simulink model "mrefrobotarm_modified_previous_y_previous_u_previous_ref"  (R2018b)
settings: Solver=FixedStepAuto  StartTime=0.0  StopTime=10  RelTol=1e-3  AbsTol=1e-6
undefined symbols (not defined in the file or in its folder): options, sfunxy2
libraries: neural x949, simulink x1
(part 22 of 31)

== system mrefrobotarm_modified_previous_y_previous_u_previous_ref/const_51traces_30x30_σ_0.0001/Layer 3/Delays 1 ==
  "p{3}" : Inport  PortDimensions=30
      mask Display: e = 0.06;c1 = [120 230 180]/255;c2 = ([120 230 180]+0)/(256+128);c3 = ([120 230 180]+128)/(256+128);patch([0 1 1 0],[0 0 1 1],c1);patch([0 1 1 1-e 1-e 0+e],[0 0 1 1-e 0+e 0+e],c2);patch([0 0 1 1-e 0+e 0+e],[0 1 1 1-e 1-e 0+e],c3);plot([0 1 1 0 0],[0 0 1 1 0]);
  mux : Mux  Inputs=1
      mask Display: e = 0.06;c1 = [120 150 230]/255;c2 = ([120 150 230]+0)/383;c3 = ([120 150 230]+128)/383;patch([0 1 1 0],[0 0 1 1],c1);patch([0 1 1 1-e 1-e 0+e],[0 0 1 1-e 0+e 0+e],c2);patch([0 0 1 1-e 0+e 0+e],[0 1 1 1-e 1-e 0+e],c3);plot([0 1 1 0 0],[0 0 1 1 0]);disp('Mux')
  "pd{3,2}" : Outport
      mask Display: e = 0.06;c1 = [120 230 180]/255;c2 = ([120 230 180]+0)/(256+128);c3 = ([120 230 180]+128)/(256+128);patch([0 1 1 0],[0 0 1 1],c1);patch([0 1 1 1-e 1-e 0+e],[0 0 1 1-e 0+e 0+e],c2);patch([0 0 1 1-e 0+e 0+e],[0 1 1 1-e 1-e 0+e],c3);plot([0 1 1 0 0],[0 0 1 1 0]);
  wires:
  "p{3}"/1 -> mux/1
  mux/1 -> "pd{3,2}"/1

== system mrefrobotarm_modified_previous_y_previous_u_previous_ref/const_51traces_30x30_σ_0.0001/Layer 3/LW{3,2} ==
  "ad{3,2}" : Inport  PortDimensions=30
      mask Display: e = 0.06;c1 = [120 230 180]/255;c2 = ([120 230 180]+0)/(256+128);c3 = ([120 230 180]+128)/(256+128);patch([0 1 1 0],[0 0 1 1],c1);patch([0 1 1 1-e 1-e 0+e],[0 0 1 1-e 0+e 0+e],c2);patch([0 0 1 1-e 0+e 0+e],[0 1 1 1-e 1-e 0+e],c3);plot([0 1 1 0 0],[0 0 1 1 0]);
  "IW{3,2}(1,:)'" : Constant  Value=[0.240977023629920295011430653175921179354190826416015625;-0.72988152363239200415279128719703294336795806884765625;-0.0304462107496987245680575284723090589977800846099853515625;-0.635040700178726158497966025606729090213775634765625;-0.612453231448408796921967223170213401317596435546875;-0.1344363308878322171846519950122456066310405731201171875;0.432506655045428123340656156869954429566860198974609375;-0.176669851226666951848898179378011263906955718994140625;-0.07557040530097362818207074042220483534038066864013671875;-0.41772110776708348822694460977800190448760986328125;0.93149781158754973997560000498197041451930999755859375;-0.31563700822511797650093967604334466159343719482421875;0.179588162001579565441033992101438343524932861328125;0.367943037247817239521197052454226650297641754150390625;0.41883849740428102936817822410375811159610748291015625;-0.50851554248389507772998285872745327651500701904296875;0.230395821119363464202223212851095013320446014404296875;-0.57517747958286757903323405116680078208446502685546875;0.71954478083832607016034899061196483671665191650390625;0.42048070720552555012972106851520948112010955810546875;-0.6720740263233346833970927036716602742671966552734375;0.183028758641015365515869461887632496654987335205078125;-0.25324226100094671121354394927038811147212982177734375;-0.0872596554170980975850824279405060224235057830810546875;-0.2750454559251604980119054744136519730091094970703125;-0.576829150618785480020278555457480251789093017578125;0.86151412289092366147968959921854548156261444091796875;-0.6458765000689965507518763843108899891376495361328125;1.0786071922365649822239674904267303645610809326171875;0.399731589161183453740022741840220987796783447265625]
      mask Display: e = 0.06;c1 = [120 150 230]/255;c2 = ([120 150 230]+0)/383;c3 = ([120 150 230]+128)/383;patch([0 1 1 0],[0 0 1 1],c1);patch([0 1 1 1-e 1-e 0+e],[0 0 1 1-e 0+e 0+e],c2);patch([0 0 1 1-e 0+e 0+e],[0 1 1 1-e 1-e 0+e],c3);plot([0 1 1 0 0],[0 0 1 1 0]);disp('weights');
  Mux : Mux  Inputs=1
      mask Display: e = 0.06;c1 = [120 150 230]/255;c2 = ([120 150 230]+0)/383;c3 = ([120 150 230]+128)/383;patch([0 1 1 0],[0 0 1 1],c1);patch([0 1 1 1-e 1-e 0+e],[0 0 1 1-e 0+e 0+e],c2);patch([0 0 1 1-e 0+e 0+e],[0 1 1 1-e 1-e 0+e],c3);plot([0 1 1 0 0],[0 0 1 1 0]);disp('Mux');
  dotprod1 : neural/Weight Functions/dotprod
  "lz{3,2}" : Outport
      mask Display: e = 0.06;c1 = [120 230 180]/255;c2 = ([120 230 180]+0)/(256+128);c3 = ([120 230 180]+128)/(256+128);patch([0 1 1 0],[0 0 1 1],c1);patch([0 1 1 1-e 1-e 0+e],[0 0 1 1-e 0+e 0+e],c2);patch([0 0 1 1-e 0+e 0+e],[0 1 1 1-e 1-e 0+e],c3);plot([0 1 1 0 0],[0 0 1 1 0]);
  wires:
  "IW{3,2}(1,:)'"/1 -> dotprod1/1
  "ad{3,2}"/1 -> dotprod1/2
  dotprod1/1 -> Mux/1
  Mux/1 -> "lz{3,2}"/1

== system mrefrobotarm_modified_previous_y_previous_u_previous_ref/const_51traces_30x30_σ_0.001/Layer 1/Delays 1 ==
  "p{1}" : Inport  PortDimensions=10
      mask Display: e = 0.06;c1 = [120 230 180]/255;c2 = ([120 230 180]+0)/(256+128);c3 = ([120 230 180]+128)/(256+128);patch([0 1 1 0],[0 0 1 1],c1);patch([0 1 1 1-e 1-e 0+e],[0 0 1 1-e 0+e 0+e],c2);patch([0 0 1 1-e 0+e 0+e],[0 1 1 1-e 1-e 0+e],c3);plot([0 1 1 0 0],[0 0 1 1 0]);
  mux : Mux  Inputs=1
      mask Display: e = 0.06;c1 = [120 150 230]/255;c2 = ([120 150 230]+0)/383;c3 = ([120 150 230]+128)/383;patch([0 1 1 0],[0 0 1 1],c1);patch([0 1 1 1-e 1-e 0+e],[0 0 1 1-e 0+e 0+e],c2);patch([0 0 1 1-e 0+e 0+e],[0 1 1 1-e 1-e 0+e],c3);plot([0 1 1 0 0],[0 0 1 1 0]);disp('Mux')
  "pd{1,1}" : Outport
      mask Display: e = 0.06;c1 = [120 230 180]/255;c2 = ([120 230 180]+0)/(256+128);c3 = ([120 230 180]+128)/(256+128);patch([0 1 1 0],[0 0 1 1],c1);patch([0 1 1 1-e 1-e 0+e],[0 0 1 1-e 0+e 0+e],c2);patch([0 0 1 1-e 0+e 0+e],[0 1 1 1-e 1-e 0+e],c3);plot([0 1 1 0 0],[0 0 1 1 0]);
  wires:
  "p{1}"/1 -> mux/1
  mux/1 -> "pd{1,1}"/1

== system mrefrobotarm_modified_previous_y_previous_u_previous_ref/const_51traces_30x30_σ_0.001/Layer 1/IW{1,1} ==
  "pd{1,1}" : Inport  PortDimensions=10
      mask Display: e = 0.06;c1 = [120 230 180]/255;c2 = ([120 230 180]+0)/(256+128);c3 = ([120 230 180]+128)/(256+128);patch([0 1 1 0],[0 0 1 1],c1);patch([0 1 1 1-e 1-e 0+e],[0 0 1 1-e 0+e 0+e],c2);patch([0 0 1 1-e 0+e 0+e],[0 1 1 1-e 1-e 0+e],c3);plot([0 1 1 0 0],[0 0 1 1 0]);
  "IW{1,1}(1,:)'" : Constant  Value=[0.88647590430992784238384274431155063211917877197265625;-1.14613055383974771217481247731484472751617431640625;0.43149650278918649792814221655135042965412139892578125;-0.3599801224142209488121579852304421365261077880859375;1.1960164258275838289335979425231926143169403076171875;-0.61109131411137285194712376323877833783626556396484375;-0.1400609285406480830626918532288982532918453216552734375;-0.5627127955935364855832858665962703526020050048828125;1.0868171814027147714654120136401616036891937255859375;0.590166554455455294458943171775899827480316162109375]
      mask Display: e = 0.06;c1 = [120 150 230]/255;c2 = ([120 150 230]+0)/383;c3 = ([120 150 230]+128)/383;patch([0 1 1 0],[0 0 1 1],c1);patch([0 1 1 1-e 1-e 0+e],[0 0 1 1-e 0+e 0+e],c2);patch([0 0 1 1-e 0+e 0+e],[0 1 1 1-e 1-e 0+e],c3);plot([0 1 1 0 0],[0 0 1 1 0]);disp('Weights');
  "IW{1,1}(10,:)'" : Constant  Value=[-1.2142966679649254135853198022232390940189361572265625;0.7923988402907820027820662289741449058055877685546875;-0.0939776780882374540571078114226111210882663726806640625;-0.43838558129977889255002310164854861795902252197265625;0.30510202260699303966617890182533301413059234619140625;0.0798827324582818409925977221064385958015918731689453125;-1.3502873847698875220402214836212806403636932373046875;-0.385994205104438770081998200112138874828815460205078125;-0.002611353880893824315478912723165194620378315448760986328125;0.5342263949565795311258398214704357087612152099609375]
      mask Display: e = 0.06;c1 = [120 150 230]/255;c2 = ([120 150 230]+0)/383;c3 = ([120 150 230]+128)/383;patch([0 1 1 0],[0 0 1 1],c1);patch([0 1 1 1-e 1-e 0+e],[0 0 1 1-e 0+e 0+e],c2);patch([0 0 1 1-e 0+e 0+e],[0 1 1 1-e 1-e 0+e],c3);plot([0 1 1 0 0],[0 0 1 1 0]);disp('Weights');
  "IW{1,1}(11,:)'" : Constant  Value=[0.52551988502623869781160692582488991320133209228515625;-1.3023156568469591576331367832608520984649658203125;-0.0716415511593599119155584276086301542818546295166015625;-0.55450379058502397011665152604109607636928558349609375;-0.230954917200865639248519300963380374014377593994140625;0.452249109231775470174596875949646346271038055419921875;-0.86426961935203916453929195995442569255828857421875;-0.9549970517556440885442725630127824842929840087890625;-0.1924050964451662071308390977719682268798351287841796875;0.10583122693447775952702016866169287823140621185302734375]
      mask Display: e = 0.06;c1 = [120 150 230]/255;c2 = ([120 150 230]+0)/383;c3 = ([120 150 230]+128)/383;patch([0 1 1 0],[0 0 1 1],c1);patch([0 1 1 1-e 1-e 0+e],[0 0 1 1-e 0+e 0+e],c2);patch([0 0 1 1-e 0+e 0+e],[0 1 1 1-e 1-e 0+e],c3);plot([0 1 1 0 0],[0 0 1 1 0]);disp('Weights');
  "IW{1,1}(12,:)'" : Constant  Value=[-0.387313692266497755500864741406985558569431304931640625;0.429686255286772678108064837942947633564472198486328125;-0.95932065522831300174999569208011962473392486572265625;-0.090550079651663784030546366921043954789638519287109375;0.5727868458286546893276636183145456016063690185546875;0.87868876198865553117656190806883387267589569091796875;-1.7317258283279617359085023053921759128570556640625;-0.8527971123216737669991971415583975613117218017578125;0.31308642872469338858110177170601673424243927001953125;0.372259712843441559204649138337117619812488555908203125]
      mask Display: e = 0.06;c1 = [120 150 230]/255;c2 = ([120 150 230]+0)/383;c3 = ([120 150 230]+128)/383;patch([0 1 1 0],[0 0 1 1],c1);patch([0 1 1 1-e 1-e 0+e],[0 0 1 1-e 0+e 0+e],c2);patch([0 0 1 1-e 0+e 0+e],[0 1 1 1-e 1-e 0+e],c3);plot([0 1 1 0 0],[0 0 1 1 0]);disp('Weights');
  "IW{1,1}(13,:)'" : Constant  Value=[-1.25614456387378492507878036121837794780731201171875;-0.5877910303392492874507979649933986365795135498046875;1.84758793112290931048846687190234661102294921875;-0.420507467934437217937926334343501366674900054931640625;-0.5430993843563971523735744995065033435821533203125;0.076738152362635203562746255556703545153141021728515625;-1.0783832881460242436588714554090984165668487548828125;0.0126228514731737927190291514989439747296273708343505859375;0.6739402421483422500614324235357344150543212890625;0.54534617577532717991317667838302440941333770751953125]
      mask Display: e = 0.06;c1 = [120 150 230]/255;c2 = ([120 150 230]+0)/383;c3 = ([120 150 230]+128)/383;patch([0 1 1 0],[0 0 1 1],c1);patch([0 1 1 1-e 1-e 0+e],[0 0 1 1-e 0+e 0+e],c2);patch([0 0 1 1-e 0+e 0+e],[0 1 1 1-e 1-e 0+e],c3);plot([0 1 1 0 0],[0 0 1 1 0]);disp('Weights');
  "IW{1,1}(14,:)'" : Constant  Value=[-0.5610919404950094335760013564140535891056060791015625;-0.054761539049275380353076769779363530687987804412841796875;1.42372282804068372996653124573640525341033935546875;-0.05361445587794340383869240440617431886494159698486328125;1.5687698740827966670252635594806633889675140380859375;-0.62361349109505581633783322104136459529399871826171875;0.281870101393739247441772022284567356109619140625;0.132740699085331648188201825178111903369426727294921875;-0.64733196498112566263927192267146892845630645751953125;-0.55118751847270852639582017218344844877719879150390625]
      mask Display: e = 0.06;c1 = [120 150 230]/255;c2 = ([120 150 230]+0)/383;c3 = ([120 150 230]+128)/383;patch([0 1 1 0],[0 0 1 1],c1);patch([0 1 1 1-e 1-e 0+e],[0 0 1 1-e 0+e 0+e],c2);patch([0 0 1 1-e 0+e 0+e],[0 1 1 1-e 1-e 0+e],c3);plot([0 1 1 0 0],[0 0 1 1 0]);disp('Weights');
  "IW{1,1}(15,:)'" : Constant  Value=[-1.9411344048006611284762357172439806163311004638671875;2.326146040891350796897540931240655481815338134765625;-0.230970377794815051597510091596632264554500579833984375;-0.0191512345205407281956144771584149566479027271270751953125;-0.05470523213543997120833495273473090492188930511474609375;-0.8832535760934174806635610366356559097766876220703125;1.1713944845459016708133503925637342035770416259765625;-0.405518430821696418409061379861668683588504791259765625;-0.1373891257194361503746193875485914759337902069091796875;-0.1887055562416380671830751225570566020905971527099609375]
      mask Display: e = 0.06;c1 = [120 150 230]/255;c2 = ([120 150 230]+0)/383;c3 = ([120 150 230]+128)/383;patch([0 1 1 0],[0 0 1 1],c1);patch([0 1 1 1-e 1-e 0+e],[0 0 1 1-e 0+e 0+e],c2);patch([0 0 1 1-e 0+e 0+e],[0 1 1 1-e 1-e 0+e],c3);plot([0 1 1 0 0],[0 0 1 1 0]);disp('Weights');
  "IW{1,1}(16,:)'" : Constant  Value=[-0.7164923870544532835680229254649020731449127197265625;-0.8690128499532681072281548040336929261684417724609375;0.331242213568548660163060048944316804409027099609375;0.476331520597255586579876762698404490947723388671875;-0.2392438611302276918468834310260717757046222686767578125;-1.648318417891640574879374980810098350048065185546875;0.6083784402561971393907924721133895218372344970703125;-0.479773713578626026521334324570489116013050079345703125;0.32137233228833517184597212690277956426143646240234375;-0.077657410543244598244427834288217127323150634765625]
      mask Display: e = 0.06;c1 = [120 150 230]/255;c2 = ([120 150 230]+0)/383;c3 = ([120 150 230]+128)/383;patch([0 1 1 0],[0 0 1 1],c1);patch([0 1 1 1-e 1-e 0+e],[0 0 1 1-e 0+e 0+e],c2);patch([0 0 1 1-e 0+e 0+e],[0 1 1 1-e 1-e 0+e],c3);plot([0 1 1 0 0],[0 0 1 1 0]);disp('Weights');
  "IW{1,1}(17,:)'" : Constant  Value=[-2.0928207094062347692897674278356134891510009765625;1.1333921124488590681522737213526852428913116455078125;0.2436558329696220936977368864972959272563457489013671875;0.57908718336795617087631171671091578900814056396484375;-0.053129695756825544294965624203541665337979793548583984375;0.82751060843652701759509682233328931033611297607421875;-0.7738951508536626722190021610003896057605743408203125;0.2119294387762725440094158102510846219956874847412109375;0.319819577337992988486092826860840432345867156982421875;0.251131352053680034774885143633582629263401031494140625]
      mask Display: e = 0.06;c1 = [120 150 230]/255;c2 = ([120 150 230]+0)/383;c3 = ([120 150 230]+128)/383;patch([0 1 1 0],[0 0 1 1],c1);patch([0 1 1 1-e 1-e 0+e],[0 0 1 1-e 0+e 0+e],c2);patch([0 0 1 1-e 0+e 0+e],[0 1 1 1-e 1-e 0+e],c3);plot([0 1 1 0 0],[0 0 1 1 0]);disp('Weights');
  "IW{1,1}(18,:)'" : Constant  Value=[-0.4122265323291178784614885444170795381069183349609375;0.73672628799896477946873574182973243296146392822265625;-0.239290661988695141371152885767514817416667938232421875;0.08962867920218543782429065913675003685057163238525390625;1.3130795126584458021312684650183655321598052978515625;0.8249569542701771229786800176952965557575225830078125;-0.5734716364476799554950048332102596759796142578125;0.32220931283260700883630534008261747658252716064453125;0.404090567428519176207402097134036011993885040283203125;0.402109996183113771461847818500245921313762664794921875]
      mask Display: e = 0.06;c1 = [120 150 230]/255;c2 = ([120 150 230]+0)/383;c3 = ([120 150 230]+128)/383;patch([0 1 1 0],[0 0 1 1],c1);patch([0 1 1 1-e 1-e 0+e],[0 0 1 1-e 0+e 0+e],c2);patch([0 0 1 1-e 0+e 0+e],[0 1 1 1-e 1-e 0+e],c3);plot([0 1 1 0 0],[0 0 1 1 0]);disp('Weights');
  "IW{1,1}(19,:)'" : Constant  Value=[-2.118850089708957273870737481047399342060089111328125;0.6347893845452656780281586179626174271106719970703125;0.97211407073288935709598490575444884598255157470703125;0.5121431870732011670810379655449651181697845458984375;-0.406246003226239216221671313178376294672489166259765625;0.94847719721738388276577325086691416800022125244140625;-0.7102564152048820300677789418841712176799774169921875;0.0811496480015026222520901910684187896549701690673828125;-0.077569687242050322506514703491120599210262298583984375;0.1878282976390456548987373253112309612333774566650390625]
      mask Display: e = 0.06;c1 = [120 150 230]/255;c2 = ([120 150 230]+0)/383;c3 = ([120 150 230]+128)/383;patch([0 1 1 0],[0 0 1 1],c1);patch([0 1 1 1-e 1-e 0+e],[0 0 1 1-e 0+e 0+e],c2);patch([0 0 1 1-e 0+e 0+e],[0 1 1 1-e 1-e 0+e],c3);plot([0 1 1 0 0],[0 0 1 1 0]);disp('Weights');
  "IW{1,1}(2,:)'" : Constant  Value=[-0.313257085634319254463520110220997594296932220458984375;0.7286897052037304423066643721540458500385284423828125;-0.5203645417886988422395688758115284144878387451171875;-0.51693659700237082343932115691131912171840667724609375;0.3651607836022439101952841156162321567535400390625;-0.64593850834349197942430009788949973881244659423828125;-0.336786483559425919853680397864081896841526031494140625;0.260117299543795976735083286257577128708362579345703125;-1.1992681308720600785733267912291921675205230712890625;-0.398556029791291288599808240178390406072139739990234375]
      mask Display: e = 0.06;c1 = [120 150 230]/255;c2 = ([120 150 230]+0)/383;c3 = ([120 150 230]+128)/383;patch([0 1 1 0],[0 0 1 1],c1);patch([0 1 1 1-e 1-e 0+e],[0 0 1 1-e 0+e 0+e],c2);patch([0 0 1 1-e 0+e 0+e],[0 1 1 1-e 1-e 0+e],c3);plot([0 1 1 0 0],[0 0 1 1 0]);disp('Weights');
  "IW{1,1}(20,:)'" : Constant  Value=[-2.325790065228988456880188095965422689914703369140625;-0.79385756422430109324750446830876171588897705078125;2.014777521227398171532740889233537018299102783203125;0.51980984727200529871282697058632038533687591552734375;-0.873647536591071638412131505901925265789031982421875;-0.297842745402778386054620796130620874464511871337890625;0.11769269572367714593585930060726241208612918853759765625;-0.009965195805270610218684623760054819285869598388671875;0.1877710921067496097069948746138834394514560699462890625;0.26877118123566756668907373750698752701282501220703125]
      mask Display: e = 0.06;c1 = [120 150 230]/255;c2 = ([120 150 230]+0)/383;c3 = ([120 150 230]+128)/383;patch([0 1 1 0],[0 0 1 1],c1);patch([0 1 1 1-e 1-e 0+e],[0 0 1 1-e 0+e 0+e],c2);patch([0 0 1 1-e 0+e 0+e],[0 1 1 1-e 1-e 0+e],c3);plot([0 1 1 0 0],[0 0 1 1 0]);disp('Weights');
  "IW{1,1}(21,:)'" : Constant  Value=[0.475027563966901933412145808688364923000335693359375;1.0297356749686847887659268963034264743328094482421875;-0.2157676398971828113371174140411312691867351531982421875;-1.03106902569636016409049261710606515407562255859375;-1.4245942055203737464097457632306031882762908935546875;0.0165937973850812346687799703204291290603578090667724609375;0.11927925766200599133615156688392744399607181549072265625;0.189034476566122766616473427347955293953418731689453125;0.69183144750120739718823870134656317532062530517578125;0.191574686569392194090966086150729097425937652587890625]
      mask Display: e = 0.06;c1 = [120 150 230]/255;c2 = ([120 150 230]+0)/383;c3 = ([120 150 230]+128)/383;patch([0 1 1 0],[0 0 1 1],c1);patch([0 1 1 1-e 1-e 0+e],[0 0 1 1-e 0+e 0+e],c2);patch([0 0 1 1-e 0+e 0+e],[0 1 1 1-e 1-e 0+e],c3);plot([0 1 1 0 0],[0 0 1 1 0]);disp('Weights');
  "IW{1,1}(22,:)'" : Constant  Value=[1.77029988058430109987284595263190567493438720703125;-1.9471924183801918584180157267837785184383392333984375;0.021924129593678239047438438547033001668751239776611328125;0.1362109015280193735630831497473991475999355316162109375;-0.90112037444176762424064008882851339876651763916015625;1.30986153869044930075915544875897467136383056640625;0.329201020828471080381660840430413372814655303955078125;-0.61721703470850297623684355130535550415515899658203125;-0.1516525428049821100362493098145932890474796295166015625;0.08554507206315191403245279389011557213962078094482421875]
      mask Display: e = 0.06;c1 = [120 150 230]/255;c2 = ([120 150 230]+0)/383;c3 = ([120 150 230]+128)/383;patch([0 1 1 0],[0 0 1 1],c1);patch([0 1 1 1-e 1-e 0+e],[0 0 1 1-e 0+e 0+e],c2);patch([0 0 1 1-e 0+e 0+e],[0 1 1 1-e 1-e 0+e],c3);plot([0 1 1 0 0],[0 0 1 1 0]);disp('Weights');
  "IW{1,1}(23,:)'" : Constant  Value=[-1.99153441779345907747256205766461789608001708984375;1.4301005486585278703159929136745631694793701171875;0.93824887701099213277444732739240862429141998291015625;-0.430803704645582208332399432038073427975177764892578125;-0.58676537144859330918933437715168111026287078857421875;1.7502962732896250042102792576770298182964324951171875;-0.67944787464199640769635379911051131784915924072265625;-0.039475618486232877391017836998798884451389312744140625;-0.09758247548192953979562247468493296764791011810302734375;0.2125958287874346874790632000440382398664951324462890625]
      mask Display: e = 0.06;c1 = [120 150 230]/255;c2 = ([120 150 230]+0)/383;c3 = ([120 150 230]+128)/383;patch([0 1 1 0],[0 0 1 1],c1);patch([0 1 1 1-e 1-e 0+e],[0 0 1 1-e 0+e 0+e],c2);patch([0 0 1 1-e 0+e 0+e],[0 1 1 1-e 1-e 0+e],c3);plot([0 1 1 0 0],[0 0 1 1 0]);disp('Weights');
  "IW{1,1}(24,:)'" : Constant  Value=[0.409743891052498809823845249411533586680889129638671875;0.371715538343925289144209500591387040913105010986328125;-0.84254512851411111906685391659266315400600433349609375;-0.38595258572140023201058056656620465219020843505859375;-1.1877493831697767401323062586016021668910980224609375;1.1652074031969019696219902471057139337062835693359375;-0.826394917437582865460399261792190372943878173828125;-0.0248924316082747461298385616146333632059395313262939453125;0.377326467362888939849341340959654189646244049072265625;0.641673097341672882265584121341817080974578857421875]
      mask Display: e = 0.06;c1 = [120 150 230]/255;c2 = ([120 150 230]+0)/383;c3 = ([120 150 230]+128)/383;patch([0 1 1 0],[0 0 1 1],c1);patch([0 1 1 1-e 1-e 0+e],[0 0 1 1-e 0+e 0+e],c2);patch([0 0 1 1-e 0+e 0+e],[0 1 1 1-e 1-e 0+e],c3);plot([0 1 1 0 0],[0 0 1 1 0]);disp('Weights');
  "IW{1,1}(25,:)'" : Constant  Value=[0.28817868868649576530316380740259774029254913330078125;-0.52882422016357022442889501689933240413665771484375;0.69738088363743055975163542825612239539623260498046875;0.366417384497668086051902491817600093781948089599609375;0.60040294518652703725791752731311134994029998779296875;0.67415561872680507260469084940268658101558685302734375;0.262363625232604091852550709518254734575748443603515625;-0.27150124742594794469141561421565711498260498046875;0.344876445354188321257282723308890126645565032958984375;0.0925003117151812492835460943751968443393707275390625]
      mask Display: e = 0.06;c1 = [120 150 230]/255;c2 = ([120 150 230]+0)/383;c3 = ([120 150 230]+128)/383;patch([0 1 1 0],[0 0 1 1],c1);patch([0 1 1 1-e 1-e 0+e],[0 0 1 1-e 0+e 0+e],c2);patch([0 0 1 1-e 0+e 0+e],[0 1 1 1-e 1-e 0+e],c3);plot([0 1 1 0 0],[0 0 1 1 0]);disp('Weights');
  "IW{1,1}(26,:)'" : Constant  Value=[-0.641978959254567715930761551135219633579254150390625;0.53519576981812078120270825820625759661197662353515625;-0.0205735159908295994757310154454899020493030548095703125;0.35448702136376908367054738846491090953350067138671875;-2.101653900721125456385607321863062679767608642578125;1.2959774861516706323527614586055278778076171875;-0.1142628343818438974022200227409484796226024627685546875;-0.076958514012763823419760456090443767607212066650390625;0.288665384838399707856382292447960935533046722412109375;0.1467535664842889164827255399359273724257946014404296875]
      mask Display: e = 0.06;c1 = [120 150 230]/255;c2 = ([120 150 230]+0)/383;c3 = ([120 150 230]+128)/383;patch([0 1 1 0],[0 0 1 1],c1);patch([0 1 1 1-e 1-e 0+e],[0 0 1 1-e 0+e 0+e],c2);patch([0 0 1 1-e 0+e 0+e],[0 1 1 1-e 1-e 0+e],c3);plot([0 1 1 0 0],[0 0 1 1 0]);disp('Weights');
  "IW{1,1}(27,:)'" : Constant  Value=[-0.346842712492006821634049629210494458675384521484375;1.0489391404250694161959245320758782327175140380859375;0.1382914780876816351895541856720228679478168487548828125;-0.820094295616564661344227715744636952877044677734375;0.311228361768038197521235588283161632716655731201171875;0.66662047703624194294746985178790055215358734130859375;-1.0279514784281611472493977998965419828891754150390625;-0.14326428827626358497582259587943553924560546875;0.0078466816705064952597314942295270157046616077423095703125;0.1358495062892683957755934898159466683864593505859375]
      mask Display: e = 0.06;c1 = [120 150 230]/255;c2 = ([120 150 230]+0)/383;c3 = ([120 150 230]+128)/383;patch([0 1 1 0],[0 0 1 1],c1);patch([0 1 1 1-e 1-e 0+e],[0 0 1 1-e 0+e 0+e],c2);patch([0 0 1 1-e 0+e 0+e],[0 1 1 1-e 1-e 0+e],c3);plot([0 1 1 0 0],[0 0 1 1 0]);disp('Weights');
  "IW{1,1}(28,:)'" : Constant  Value=[-0.4092389907150406624936067601083777844905853271484375;0.199356444802080812195299586164765059947967529296875;-0.8679224416722337576146628634887747466564178466796875;0.1778152623480658556243128032292588613927364349365234375;0.370722099273408878250535281040356494486331939697265625;-0.4384221042767595388767176700639538466930389404296875;-1.25836650250711290510707840439863502979278564453125;-0.463729863974594980202681426817434839904308319091796875;-0.70914896631661294978954401813098229467868804931640625;-0.6337029351151948208809017160092480480670928955078125]
      mask Display: e = 0.06;c1 = [120 150 230]/255;c2 = ([120 150 230]+0)/383;c3 = ([120 150 230]+128)/383;patch([0 1 1 0],[0 0 1 1],c1);patch([0 1 1 1-e 1-e 0+e],[0 0 1 1-e 0+e 0+e],c2);patch([0 0 1 1-e 0+e 0+e],[0 1 1 1-e 1-e 0+e],c3);plot([0 1 1 0 0],[0 0 1 1 0]);disp('Weights');
  "IW{1,1}(29,:)'" : Constant  Value=[0.335226811361067078554043519034166820347309112548828125;-0.75241868216664775648183649536804296076297760009765625;0.449495605580200463524676024462678469717502593994140625;-0.344021508317923885300615438609384000301361083984375;-0.2411629842875398221924143626893055625259876251220703125;0.044766518318397639786265784778152010403573513031005859375;-0.733518664383499885417450059321708977222442626953125;-0.442157524460116080344818101366399787366390228271484375;-0.2653628725454808545691776089370250701904296875;0.166311289604483547588387182258884422481060028076171875]
      mask Display: e = 0.06;c1 = [120 150 230]/255;c2 = ([120 150 230]+0)/383;c3 = ([120 150 230]+128)/383;patch([0 1 1 0],[0 0 1 1],c1);patch([0 1 1 1-e 1-e 0+e],[0 0 1 1-e 0+e 0+e],c2);patch([0 0 1 1-e 0+e 0+e],[0 1 1 1-e 1-e 0+e],c3);plot([0 1 1 0 0],[0 0 1 1 0]);disp('Weights');
  "IW{1,1}(3,:)'" : Constant  Value=[-0.484196594281250114466530476420302875339984893798828125;0.06706481367172108243313033426602487452328205108642578125;0.30414745073247939632921088559669442474842071533203125;-0.1038035640911204871006390249021933414041996002197265625;0.017392390907732806215602039401346701197326183319091796875;-0.312430763935094113481483191208099015057086944580078125;0.86849989792999304771825563875609077513217926025390625;-1.1171188331280148542390406873892061412334442138671875;-0.70116344417634757224533359476481564342975616455078125;-0.340886907428760654870103508073952980339527130126953125]
      mask Display: e = 0.06;c1 = [120 150 230]/255;c2 = ([120 150 230]+0)/383;c3 = ([120 150 230]+128)/383;patch([0 1 1 0],[0 0 1 1],c1);patch([0 1 1 1-e 1-e 0+e],[0 0 1 1-e 0+e 0+e],c2);patch([0 0 1 1-e 0+e 0+e],[0 1 1 1-e 1-e 0+e],c3);plot([0 1 1 0 0],[0 0 1 1 0]);disp('Weights');
  "IW{1,1}(30,:)'" : Constant  Value=[0.91664388852396161411206776392646133899688720703125;-0.352775808983562921827825675791245885193347930908203125;-0.79624903699780780197414742360706441104412078857421875;0.368549074207838389671820777948596514761447906494140625;0.69310017374494392594641567484359256923198699951171875;1.157399249135311780634083334007300436496734619140625;-0.652288700590936354473114988650195300579071044921875;0.0022329667532263626494870578653717529959976673126220703125;-0.87044682745007129209824370263959281146526336669921875;-0.326676834919193248563118459060206077992916107177734375]
      mask Display: e = 0.06;c1 = [120 150 230]/255;c2 = ([120 150 230]+0)/383;c3 = ([120 150 230]+128)/383;patch([0 1 1 0],[0 0 1 1],c1);patch([0 1 1 1-e 1-e 0+e],[0 0 1 1-e 0+e 0+e],c2);patch([0 0 1 1-e 0+e 0+e],[0 1 1 1-e 1-e 0+e],c3);plot([0 1 1 0 0],[0 0 1 1 0]);disp('Weights');
  "IW{1,1}(4,:)'" : Constant  Value=[-0.73917669251087858572901723164250142872333526611328125;0.29750193229649390946889297993038780987262725830078125;0.0194796061829275168886255187317146919667720794677734375;-0.6212224566058843766569452782277949154376983642578125;0.1550472028193648210692145994471502490341663360595703125;-0.69882316200475147471848913482972420752048492431640625;-0.3034536820713118476788849875447340309619903564453125;-0.9396860752657953952393654617480933666229248046875;-0.1677193169817949580657767683078418485820293426513671875;-0.2332745208501280920199150159533019177615642547607421875]
      mask Display: e = 0.06;c1 = [120 150 230]/255;c2 = ([120 150 230]+0)/383;c3 = ([120 150 230]+128)/383;patch([0 1 1 0],[0 0 1 1],c1);patch([0 1 1 1-e 1-e 0+e],[0 0 1 1-e 0+e 0+e],c2);patch([0 0 1 1-e 0+e 0+e],[0 1 1 1-e 1-e 0+e],c3);plot([0 1 1 0 0],[0 0 1 1 0]);disp('Weights');
  "IW{1,1}(5,:)'" : Constant  Value=[0.72639456932832613400563559480360709130764007568359375;-0.1487651637893023515157864267166587524116039276123046875;0.344632208768709258350781965418718755245208740234375;-0.0283082517696422418518320540670174523256719112396240234375;-2.872807326397399219075623477692715823650360107421875;1.321416533064848408685065805912017822265625;-0.08833085320734089529448596067595644854009151458740234375;1.316776194184606563197803552611730992794036865234375;-0.57331943196846613108874635145184583961963653564453125;-0.1516451874049625503371174772837548516690731048583984375]
      mask Display: e = 0.06;c1 = [120 150 230]/255;c2 = ([120 150 230]+0)/383;c3 = ([120 150 230]+128)/383;patch([0 1 1 0],[0 0 1 1],c1);patch([0 1 1 1-e 1-e 0+e],[0 0 1 1-e 0+e 0+e],c2);patch([0 0 1 1-e 0+e 0+e],[0 1 1 1-e 1-e 0+e],c3);plot([0 1 1 0 0],[0 0 1 1 0]);disp('Weights');
  "IW{1,1}(6,:)'" : Constant  Value=[-0.2806642788954218925567829501233063638210296630859375;0.035971273126059542801780111176412901841104030609130859375;0.403392500150154764693155584609485231339931488037109375;-0.2814843193630849338404686932335607707500457763671875;1.3327685960310924340177507474436424672603607177734375;1.3585988831978854651794108576723374426364898681640625;-0.9051173289101817065471777823404408991336822509765625;0.006340869953782540639763976031417769263498485088348388671875;-0.4941369066982936875120913100545294582843780517578125;0.00644011132269183862730788092676448286511003971099853515625]
      mask Display: e = 0.06;c1 = [120 150 230]/255;c2 = ([120 150 230]+0)/383;c3 = ([120 150 230]+128)/383;patch([0 1 1 0],[0 0 1 1],c1);patch([0 1 1 1-e 1-e 0+e],[0 0 1 1-e 0+e 0+e],c2);patch([0 0 1 1-e 0+e 0+e],[0 1 1 1-e 1-e 0+e],c3);plot([0 1 1 0 0],[0 0 1 1 0]);disp('Weights');
  "IW{1,1}(7,:)'" : Constant  Value=[2.0999248308277511654296176857315003871917724609375;-1.7466213019937735229092368172132410109043121337890625;-0.33257481537707478391752147217630408704280853271484375;0.0297386375753464250737412299940842785872519016265869140625;0.41413945097893656299703479817253537476062774658203125;-0.6293077512855786981305072913528420031070709228515625;-0.62516732654952755776633921414031647145748138427734375;0.6510572128186122853321649017743766307830810546875;0.6358017255818200208494772596168331801891326904296875;0.274109739742171398813042060282896272838115692138671875]
      mask Display: e = 0.06;c1 = [120 150 230]/255;c2 = ([120 150 230]+0)/383;c3 = ([120 150 230]+128)/383;patch([0 1 1 0],[0 0 1 1],c1);patch([0 1 1 1-e 1-e 0+e],[0 0 1 1-e 0+e 0+e],c2);patch([0 0 1 1-e 0+e 0+e],[0 1 1 1-e 1-e 0+e],c3);plot([0 1 1 0 0],[0 0 1 1 0]);disp('Weights');
  "IW{1,1}(8,:)'" : Constant  Value=[-0.456346391158764574935702285074512474238872528076171875;2.076682640874107477202414884231984615325927734375;-1.6400960680157703475146035998477600514888763427734375;-0.22963076285644934415586249087937176227569580078125;-0.64460129655188069808247064429451711475849151611328125;0.143288671084537799771396748838014900684356689453125;-0.97887162962283114087114199719508178532123565673828125;0.1537220951208864427872669011776451952755451202392578125;0.81526584872772211998182001480017788708209991455078125;0.5430607112901248978431567593361251056194305419921875]
      mask Display: e = 0.06;c1 = [120 150 230]/255;c2 = ([120 150 230]+0)/383;c3 = ([120 150 230]+128)/383;patch([0 1 1 0],[0 0 1 1],c1);patch([0 1 1 1-e 1-e 0+e],[0 0 1 1-e 0+e 0+e],c2);patch([0 0 1 1-e 0+e 0+e],[0 1 1 1-e 1-e 0+e],c3);plot([0 1 1 0 0],[0 0 1 1 0]);disp('Weights');
  "IW{1,1}(9,:)'" : Constant  Value=[-0.136136085133208017960981806027120910584926605224609375;0.1096753961203410232538857371764606796205043792724609375;-0.295419448817430485565438402772997505962848663330078125;0.1527498880060141062120493415932287462055683135986328125;-1.3508829661000982813590098885470069944858551025390625;-0.299911280031890437047792374869459308683872222900390625;-0.423561116920596336665738590454566292464733123779296875;0.5347165945350138560598907133680768311023712158203125;-0.7334392311239026351898928623995743691921234130859375;-0.00606445375883311009468368268926496966741979122161865234375]
      mask Display: e = 0.06;c1 = [120 150 230]/255;c2 = ([120 150 230]+0)/383;c3 = ([120 150 230]+128)/383;patch([0 1 1 0],[0 0 1 1],c1);patch([0 1 1 1-e 1-e 0+e],[0 0 1 1-e 0+e 0+e],c2);patch([0 0 1 1-e 0+e 0+e],[0 1 1 1-e 1-e 0+e],c3);plot([0 1 1 0 0],[0 0 1 1 0]);disp('Weights');
  Mux : Mux  Inputs=30
      mask Display: e = 0.06;c1 = [120 150 230]/255;c2 = ([120 150 230]+0)/383;c3 = ([120 150 230]+128)/383;patch([0 1 1 0],[0 0 1 1],c1);patch([0 1 1 1-e 1-e 0+e],[0 0 1 1-e 0+e 0+e],c2);patch([0 0 1 1-e 0+e 0+e],[0 1 1 1-e 1-e 0+e],c3);plot([0 1 1 0 0],[0 0 1 1 0]);disp('Mux');
  dotprod{1..30} (30 alike) : neural/Weight Functions/dotprod
  "iz{1,1}" : Outport
      mask Display: e = 0.06;c1 = [120 230 180]/255;c2 = ([120 230 180]+0)/(256+128);c3 = ([120 230 180]+128)/(256+128);patch([0 1 1 0],[0 0 1 1],c1);patch([0 1 1 1-e 1-e 0+e],[0 0 1 1-e 0+e 0+e],c2);patch([0 0 1 1-e 0+e 0+e],[0 1 1 1-e 1-e 0+e],c3);plot([0 1 1 0 0],[0 0 1 1 0]);
  wires:
  "IW{1,1}(1,:)'"/1 -> dotprod1/1
  "pd{1,1}"/1 -> dotprod1/2, dotprod2/2, dotprod3/2, dotprod4/2, dotprod5/2, dotprod6/2, dotprod7/2, dotprod8/2, dotprod9/2, dotprod10/2, dotprod11/2, dotprod12/2, dotprod13/2, dotprod14/2, dotprod15/2, dotprod16/2, dotprod17/2, dotprod18/2, dotprod19/2, dotprod20/2, dotprod21/2, dotprod22/2, dotprod23/2, dotprod24/2, dotprod25/2, dotprod26/2, dotprod27/2, dotprod28/2, dotprod29/2, dotprod30/2
  dotprod1/1 -> Mux/1
  "IW{1,1}(2,:)'"/1 -> dotprod2/1
  dotprod2/1 -> Mux/2
  "IW{1,1}(3,:)'"/1 -> dotprod3/1
  dotprod3/1 -> Mux/3
  "IW{1,1}(4,:)'"/1 -> dotprod4/1
  dotprod4/1 -> Mux/4
  "IW{1,1}(5,:)'"/1 -> dotprod5/1
  dotprod5/1 -> Mux/5
  "IW{1,1}(6,:)'"/1 -> dotprod6/1
  dotprod6/1 -> Mux/6
  "IW{1,1}(7,:)'"/1 -> dotprod7/1
  dotprod7/1 -> Mux/7
  "IW{1,1}(8,:)'"/1 -> dotprod8/1
  dotprod8/1 -> Mux/8
  "IW{1,1}(9,:)'"/1 -> dotprod9/1
  dotprod9/1 -> Mux/9
  "IW{1,1}(10,:)'"/1 -> dotprod10/1
  dotprod10/1 -> Mux/10
  "IW{1,1}(11,:)'"/1 -> dotprod11/1
  dotprod11/1 -> Mux/11
  "IW{1,1}(12,:)'"/1 -> dotprod12/1
  dotprod12/1 -> Mux/12
  "IW{1,1}(13,:)'"/1 -> dotprod13/1
  dotprod13/1 -> Mux/13
  "IW{1,1}(14,:)'"/1 -> dotprod14/1
  dotprod14/1 -> Mux/14
  "IW{1,1}(15,:)'"/1 -> dotprod15/1
  dotprod15/1 -> Mux/15
  "IW{1,1}(16,:)'"/1 -> dotprod16/1
  dotprod16/1 -> Mux/16
  "IW{1,1}(17,:)'"/1 -> dotprod17/1
  dotprod17/1 -> Mux/17
  "IW{1,1}(18,:)'"/1 -> dotprod18/1
  dotprod18/1 -> Mux/18
  "IW{1,1}(19,:)'"/1 -> dotprod19/1
  dotprod19/1 -> Mux/19
  "IW{1,1}(20,:)'"/1 -> dotprod20/1
  dotprod20/1 -> Mux/20
  "IW{1,1}(21,:)'"/1 -> dotprod21/1
  dotprod21/1 -> Mux/21
  "IW{1,1}(22,:)'"/1 -> dotprod22/1
  dotprod22/1 -> Mux/22
  "IW{1,1}(23,:)'"/1 -> dotprod23/1
  dotprod23/1 -> Mux/23
  "IW{1,1}(24,:)'"/1 -> dotprod24/1
  dotprod24/1 -> Mux/24
  "IW{1,1}(25,:)'"/1 -> dotprod25/1
  dotprod25/1 -> Mux/25
  "IW{1,1}(26,:)'"/1 -> dotprod26/1
  dotprod26/1 -> Mux/26
  "IW{1,1}(27,:)'"/1 -> dotprod27/1
  dotprod27/1 -> Mux/27
  "IW{1,1}(28,:)'"/1 -> dotprod28/1
  dotprod28/1 -> Mux/28
  "IW{1,1}(29,:)'"/1 -> dotprod29/1
  dotprod29/1 -> Mux/29
  "IW{1,1}(30,:)'"/1 -> dotprod30/1
  dotprod30/1 -> Mux/30
  Mux/1 -> "iz{1,1}"/1

== system mrefrobotarm_modified_previous_y_previous_u_previous_ref/const_51traces_30x30_σ_0.001/Layer 2/Delays 1 ==
  "p{2}" : Inport  PortDimensions=30
      mask Display: e = 0.06;c1 = [120 230 180]/255;c2 = ([120 230 180]+0)/(256+128);c3 = ([120 230 180]+128)/(256+128);patch([0 1 1 0],[0 0 1 1],c1);patch([0 1 1 1-e 1-e 0+e],[0 0 1 1-e 0+e 0+e],c2);patch([0 0 1 1-e 0+e 0+e],[0 1 1 1-e 1-e 0+e],c3);plot([0 1 1 0 0],[0 0 1 1 0]);
  mux : Mux  Inputs=1
      mask Display: e = 0.06;c1 = [120 150 230]/255;c2 = ([120 150 230]+0)/383;c3 = ([120 150 230]+128)/383;patch([0 1 1 0],[0 0 1 1],c1);patch([0 1 1 1-e 1-e 0+e],[0 0 1 1-e 0+e 0+e],c2);patch([0 0 1 1-e 0+e 0+e],[0 1 1 1-e 1-e 0+e],c3);plot([0 1 1 0 0],[0 0 1 1 0]);disp('Mux')
  "pd{2,1}" : Outport
      mask Display: e = 0.06;c1 = [120 230 180]/255;c2 = ([120 230 180]+0)/(256+128);c3 = ([120 230 180]+128)/(256+128);patch([0 1 1 0],[0 0 1 1],c1);patch([0 1 1 1-e 1-e 0+e],[0 0 1 1-e 0+e 0+e],c2);patch([0 0 1 1-e 0+e 0+e],[0 1 1 1-e 1-e 0+e],c3);plot([0 1 1 0 0],[0 0 1 1 0]);
  wires:
  "p{2}"/1 -> mux/1
  mux/1 -> "pd{2,1}"/1
